simulink model "modelling_with_standard_blocks"  (R2018b)
settings: Solver=VariableStepAuto  StartTime=0.0  StopTime=10.0  RelTol=1e-3
settings Model: Creator=0x6f736f646f  LastModifiedBy=0x6f736f646f

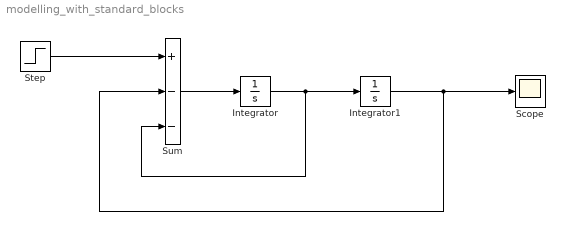
== system modelling_with_standard_blocks ==
  Integrator : Integrator
  Integrator1 : Integrator
  Scope : Scope
  Step : Step  Before=0.1  SampleTime=15
  Sum : Sum  Inputs=+--
  wires:
  Step/1 -> Sum/1
  Sum/1 -> Integrator/1
  Integrator/1 -> Sum/3, Integrator1/1
  Integrator1/1 -> Sum/2, Scope/1
